simulink model "skipper_lqr"  (R2024b)
settings: Solver=FixedStepAuto  StartTime=0.0  StopTime=20  RelTol=1e-3
libraries: matrix_library x2, aerolibanimutils x1, dspinverses x1
settings Model: Creator=nehir  LastModifiedBy=nehir
settings OptimizationCC: OptimizeBlockIOStorage=off  OptimizeDataStoreBuffers=off  BusAssignmentInplaceUpdate=off
settings DebuggingCC: SFUnexpectedBacktrackingDiag=warning  SFNoUnconditionalDefaultTransitionDiag=warning
settings RTWCC: GenerateReport=on  BuildConfiguration=Debug  LaunchReport=on
settings CodeAppCC: ForceParamTrailComments=on  MATLABSourceComments=on  EnableCustomComments=on
settings GRTTargetCC: CombineSignalStateStructs=on  SupportVariableSizeSignals=on  MultiInstanceErrorCode=Warning

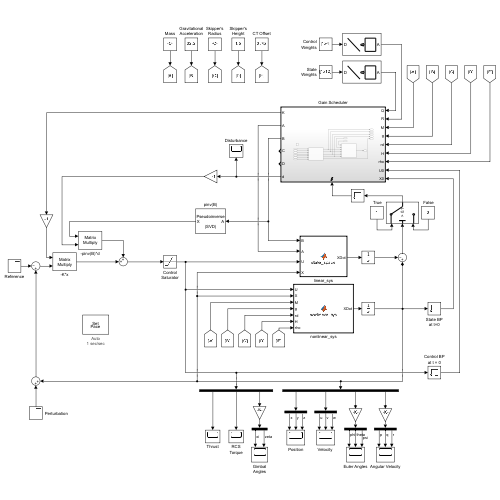
[thumbnail: Simulink's stored preview of the top-level diagram]
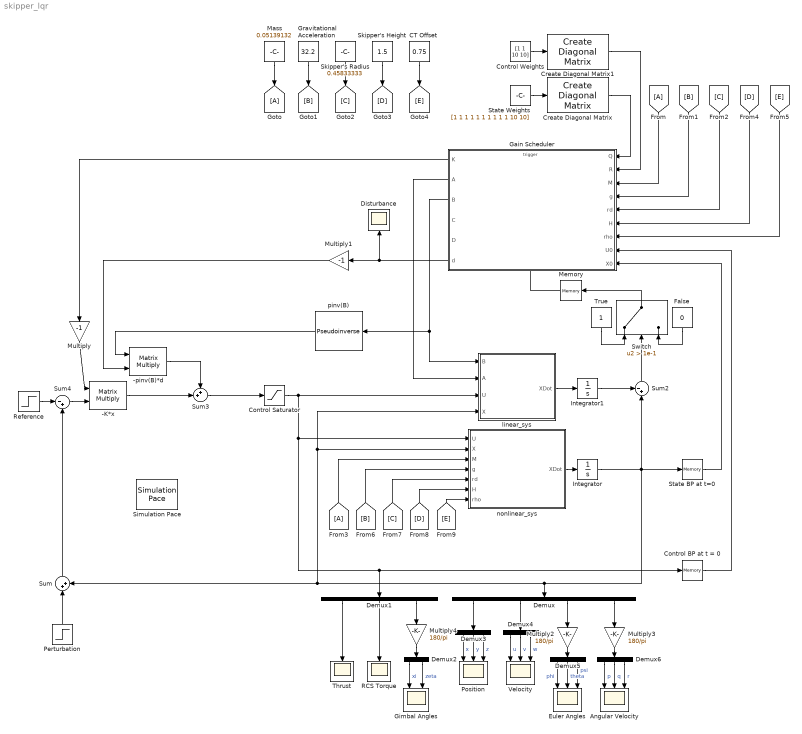
== system skipper_lqr ==
  " False" : Constant  Value=0
  " True" : Constant
  -K*x : Product  Multiplication=Matrix(*)
  -pinv(B)*d : Product  Multiplication=Matrix(*)
  Angular Velocity : Scope  NumInputPorts=3
  CT Offset : Constant  Value=0.75
  Control Saturator : Saturate  UpperLimit=[2.2 pi/2 pi/18 pi/18]'  LowerLimit=[0 -pi/2 -pi/18 -pi/18]'
  Control Weights : Constant  Value=[1 1 10 10]
  Control BP at t = 0 : Memory  InitialCondition=[10 1 0 0]'
  Create Diagonal Matrix : matrix_library/Create Diagonal Matrix
      settings: LibrarySourceBlock=|
      | simulink/Matrix
      | Operations/Create Diagonal
      | Matrix
  Create Diagonal Matrix1 : matrix_library/Create Diagonal Matrix
      settings: LibrarySourceBlock=|
      | simulink/Matrix
      | Operations/Create Diagonal
      | Matrix
  Demux : Demux  Outputs=[3 3 3 3]
  Demux1 : Demux  Outputs=[1 1 2]
  Demux2 : Demux  Outputs=[1 1]
  Demux{3..6} (4 alike) : Demux  Outputs=[1 1 1]
  Disturbance : Scope
  Euler Angles : Scope  NumInputPorts=3
  From : From
  From3 : From
  Gain Scheduler : Subsystem  TreatAsAtomicUnit=on
  Gimbal Angles : Scope  NumInputPorts=2
  Goto : Goto
  Gravitational Acceleration : Constant  Value=32.2
  Integrator : Integrator  InitialCondition=[0 0 0 0 0 0 0 0 0 0 0 0]'
  Integrator1 : Integrator  InitialCondition=[0 0 0 0 0 0 0 0 0 0 0 0]'
  Mass : Constant  Value=0.05139132
  Memory : Memory  InitialCondition=1
  Multiply : Gain  Gain=-1
  Multiply1 : Gain  Gain=-1
  Multiply2 : Gain  Gain=180/pi
  Multiply3 : Gain  Gain=180/pi
  Multiply4 : Gain  Gain=180/pi
  Perturbation : Step  Time=0.1  Before=[0 0 0 0 0 0 0 0 0 0 0 0]'  After=[0 0 0 0 0 0 0 0 0 0 0 0]'  SampleTime=0
  Position : Scope  NumInputPorts=3
  RCS Torque : Scope
  Reference : Step  Before=[0 0 0 0 0 0 0 0 0 0 0 0]'  After=[5 5 5 0 0 0 0 0 0 0 0 0]'  SampleTime=0
  Simulation Pace : aerolibanimutils/Simulation Pace  SimulationPace=1  SleepMode=Auto  OutputPaceError=off  SampleTime=1/30
  Skipper's Height : Constant  Value=1.5
  Skipper's Radius : Constant  Value=0.45833333
  State Weights : Constant  Value=[1 1 1 1 1 1 1 1 1 1 10 10]
  State BP at t=0 : Memory  InitialCondition=[0 0 0 0 0 0 0 0 0 0 0 0]'
  Sum : Sum  Inputs=|++
  Sum2 : Sum  Inputs=-+|
  Sum3 : Sum  Inputs=++|
  Sum4 : Sum  Inputs=|-+
  Switch : Switch  Criteria=u2 > Threshold  Threshold=1e-1  ZeroCross=off  SaturateOnIntegerOverflow=off  InputSameDT=off
  Thrust : Scope
  "Velocity " : Scope  NumInputPorts=3
  linear_sys : MATLAB Function  TreatAsAtomicUnit=on
  nonlinear_sys : MATLAB Function  TreatAsAtomicUnit=on
  pinv(B) : dspinverses/Pseudoinverse  wanterr=off  SimulateUsing=Interpreted execution
  wires:
  Demux1/2 -> RCS Torque/1
  Demux1/1 -> Thrust/1
  Demux/1 -> Demux3/1
  Demux/2 -> Demux4/1
  Demux/3 -> Multiply2/1
  Demux/4 -> Multiply3/1
  Demux1/3 -> Multiply4/1
  Demux2/1 -> Gimbal Angles/1  "xi"
  Demux2/2 -> Gimbal Angles/2  "zeta"
  Demux3/1 -> Position/1  "x"
  Demux3/3 -> Position/3  "z"
  Demux4/1 -> "Velocity "/1  "u"
  Demux4/2 -> "Velocity "/2  "v"
  Demux4/3 -> "Velocity "/3  "w"
  Demux5/1 -> Euler Angles/1  "phi"
  Demux5/2 -> Euler Angles/2  "theta"
  Demux5/3 -> Euler Angles/3  "psi"
  Demux3/2 -> Position/2  "y"
  Demux6/1 -> Angular Velocity/1  "p"
  Demux6/2 -> Angular Velocity/2  "q"
  Demux6/3 -> Angular Velocity/3  "r"
  nonlinear_sys/1(XDot) -> Integrator/1
  Sum4/1 -> -K*x/2
  Sum2/1 -> Switch/2
  linear_sys/1(XDot) -> Integrator1/1
  Integrator1/1 -> Sum2/1
  State Weights/1 -> Create Diagonal Matrix/1
  Control Weights/1 -> Create Diagonal Matrix1/1
  Multiply/1 -> -K*x/1
  pinv(B)/1 -> -pinv(B)*d/1
  Multiply1/1 -> -pinv(B)*d/2
  Gain Scheduler/6(d) -> Disturbance/1, Multiply1/1
  Gain Scheduler/3(B) -> pinv(B)/1, linear_sys/1(B)
  Gain Scheduler/1(K) -> Multiply/1
  Switch/1 -> Memory/1
  " True"/1 -> Switch/1
  " False"/1 -> Switch/3
  Create Diagonal Matrix/1 -> Gain Scheduler/1(Q)
  Create Diagonal Matrix1/1 -> Gain Scheduler/2(R)
  Gain Scheduler/2(A) -> linear_sys/2(A)
  Integrator/1 -> Demux/1, nonlinear_sys/2(X), linear_sys/4(X), Sum/2, State BP at t=0/1, Sum2/2
  Control BP at t = 0/1 -> Gain Scheduler/8(U0)
  State BP at t=0/1 -> Gain Scheduler/9(X0)
  Memory/1 -> Gain Scheduler/Trigger
  -K*x/1 -> Sum3/2
  Control Saturator/1 -> linear_sys/3(U), nonlinear_sys/1(U), Demux1/1, Control BP at t = 0/1
  Multiply2/1 -> Demux5/1
  Multiply3/1 -> Demux6/1
  Multiply4/1 -> Demux2/1
  [E] -> nonlinear_sys/7(rho)
  [B] -> nonlinear_sys/4(g)
  [D] -> nonlinear_sys/6(H)
  [C] -> nonlinear_sys/5(rd)
  From3/1 -> nonlinear_sys/3(M)
  CT Offset/1 -> [E]
  Gravitational Acceleration/1 -> [B]
  Mass/1 -> Goto/1
  Skipper's Height/1 -> [D]
  Skipper's Radius/1 -> [C]
  [D] -> Gain Scheduler/6(H)
  [B] -> Gain Scheduler/4(g)
  [C] -> Gain Scheduler/5(rd)
  From/1 -> Gain Scheduler/3(M)
  [E] -> Gain Scheduler/7(rho)
  Reference/1 -> Sum4/1
  Sum/1 -> Sum4/2
  Perturbation/1 -> Sum/1
  Sum3/1 -> Control Saturator/1
  -pinv(B)*d/1 -> Sum3/1

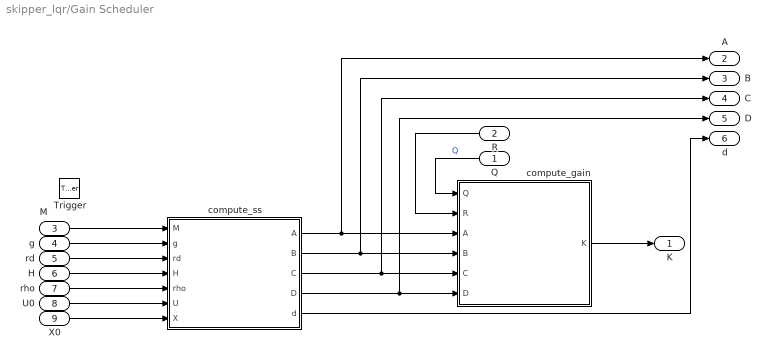
== system skipper_lqr/Gain Scheduler ==
  Q : Inport
  R : Inport  Port=2
  M : Inport  Port=3
  g : Inport  Port=4
  rd : Inport  Port=5
  H : Inport  Port=6
  rho : Inport  Port=7
  U0 : Inport  Port=8
  X0 : Inport  Port=9
  Trigger : TriggerPort  VariantControl=(inherit)  ZeroCross=off  InitialTriggerSignalState=negative
  compute_gain : MATLAB Function  TreatAsAtomicUnit=on
  compute_ss : MATLAB Function  TreatAsAtomicUnit=on
  K : Outport
  A : Outport  Port=2
  B : Outport  Port=3
  C : Outport  Port=4
  D : Outport  Port=5
  d : Outport  Port=6
  wires:
  M/1 -> compute_ss/1(M)
  R/1 -> compute_gain/2(R)
  Q/1 -> compute_gain/1(Q)  "Q"
  U0/1 -> compute_ss/6(U)
  rho/1 -> compute_ss/5(rho)
  H/1 -> compute_ss/4(H)
  rd/1 -> compute_ss/3(rd)
  g/1 -> compute_ss/2(g)
  X0/1 -> compute_ss/7(X)
  compute_ss/1(A) -> A/1, compute_gain/3(A)
  compute_ss/2(B) -> B/1, compute_gain/4(B)
  compute_ss/3(C) -> compute_gain/5(C), C/1
  compute_ss/4(D) -> compute_gain/6(D), D/1
  compute_ss/5(d) -> d/1
  compute_gain/1(K) -> K/1

== matlab function skipper_lqr/Gain Scheduler/compute_ss ==
  data: M input; g input; rd input; H input; rho input; U input; X input; A output; B output; C output; D output; d output
function [A, B, C, D, d] = compute_ss(M, g, rd, H, rho, U, X)
% ________________________________________________________________________
%
%                           STATE SPACE MATRICES
% ________________________________________________________________________
% 
% BY:       FLORIDA ROCKET LAB - GNC SUBTEAM
% EDITORS:  N. HIRSCH, L. DAPP
% DATE:     1/20/25
%
% OVERVIEW: Calculates A, B, C, D, matices for use in a state
% space Simulink model and LQR controller as well as the disturbance, d.

    %save('basepoints.mat', 'U', 'X')
    
    % Calculate rotational inertias in body frame.
    Ixx = M*rd^2/2;
    Iyy = M*(3*rd^2+H^2)/12;
    Izz = Iyy;
    
    % Initialize state space matricies. Since they are sparse simply use zeros
    % and then input non-zero terms individually.
    % x = [x y z u v w phi theta psi p q r]
    % u = [T tauR xi zeta]
    x0 = X(1);
    y0 = X(2);
    z0 = X(3);
    u0 = X(4);
    v0 = X(5);
    w0 = X(6);
    phi0 = X(7);
    theta0 = X(8);
    psi0 = X(9);
    p0 = X(10);
    q0 = X(11);
    r0 = X(12);

    T0 = U(1);
    tauR0 = U(2);
    xi0 = U(3);
    zeta0 = U(4);

    % BEGIN "A"; Do not modify this. The python script looks for this line.
    A = [
        0 0 0 cos(psi0)*cos(theta0) sin(phi0)*sin(theta0)*cos(psi0)-sin(psi0)*cos(phi0) sin(phi0)*sin(psi0)+sin(theta0)*cos(phi0)*cos(psi0) v0*sin(phi0)*sin(psi0)+v0*sin(theta0)*cos(phi0)*cos(psi0)-w0*sin(phi0)*sin(theta0)*cos(psi0)+w0*sin(psi0)*cos(phi0) -u0*sin(theta0)*cos(psi0)+v0*sin(phi0)*cos(psi0)*cos(theta0)+w0*cos(phi0)*cos(psi0)*cos(theta0) -u0*sin(psi0)*cos(theta0)-v0*sin(phi0)*sin(psi0)*sin(theta0)-v0*cos(phi0)*cos(psi0)+w0*sin(phi0)*cos(psi0)-w0*sin(psi0)*sin(theta0)*cos(phi0) 0 0 0;
        0 0 0 sin(psi0)*cos(theta0) sin(phi0)*sin(psi0)*sin(theta0)+cos(phi0)*cos(psi0) -sin(phi0)*cos(psi0)+sin(psi0)*sin(theta0)*cos(phi0) -v0*sin(phi0)*cos(psi0)+v0*sin(psi0)*sin(theta0)*cos(phi0)-w0*sin(phi0)*sin(psi0)*sin(theta0)-w0*cos(phi0)*cos(psi0) -u0*sin(psi0)*sin(theta0)+v0*sin(phi0)*sin(psi0)*cos(theta0)+w0*sin(psi0)*cos(phi0)*cos(theta0) u0*cos(psi0)*cos(theta0)+v0*sin(phi0)*sin(theta0)*cos(psi0)-v0*sin(psi0)*cos(phi0)+w0*sin(phi0)*sin(psi0)+w0*sin(theta0)*cos(phi0)*cos(psi0) 0 0 0;
        0 0 0 -sin(theta0) sin(phi0)*cos(theta0) cos(phi0)*cos(theta0) v0*cos(phi0)*cos(theta0)-w0*sin(phi0)*cos(theta0) -u0*cos(theta0)-v0*sin(phi0)*sin(theta0)-w0*sin(theta0)*cos(phi0) 0 0 0 0;
        0 0 0 0 r0 -q0 0 g*sin(theta0)*cos(psi0) g*sin(psi0)*cos(theta0) 0 -w0 v0;
        0 0 0 -r0 0 p0 -g*sin(phi0)*sin(psi0)-g*sin(theta0)*cos(phi0)*cos(psi0) -g*sin(phi0)*cos(psi0)*cos(theta0) g*sin(phi0)*sin(psi0)*sin(theta0)+g*cos(phi0)*cos(psi0) w0 0 -u0;
        0 0 0 q0 -p0 0 g*sin(phi0)*sin(theta0)*cos(psi0)-g*sin(psi0)*cos(phi0) -g*cos(phi0)*cos(psi0)*cos(theta0) -g*sin(phi0)*cos(psi0)+g*sin(psi0)*sin(theta0)*cos(phi0) -v0 u0 0;
        0 0 0 0 0 0 q0*cos(phi0)*tan(theta0)-r0*sin(phi0)*tan(theta0) q0*sin(phi0)*tan(theta0)^2+q0*sin(phi0)+r0*cos(phi0)*tan(theta0)^2+r0*cos(phi0) 0 1 sin(phi0)*tan(theta0) cos(phi0)*tan(theta0);
        0 0 0 0 0 0 -q0*sin(phi0)-r0*cos(phi0) 0 0 0 cos(phi0) -sin(phi0);
        0 0 0 0 0 0 q0*cos(phi0)/cos(theta0)-r0*sin(phi0)/cos(theta0) q0*sin(phi0)*sin(theta0)/cos(theta0)^2+r0*sin(theta0)*cos(phi0)/cos(theta0)^2 0 0 sin(phi0)/cos(theta0) cos(phi0)/cos(theta0);
        0 0 0 0 0 0 0 0 0 0 Iyy*r0/Ixx-Izz*r0/Ixx Iyy*q0/Ixx-Izz*q0/Ixx;
        0 0 0 0 0 0 0 0 0 -Ixx*r0/Iyy+Izz*r0/Iyy 0 -Ixx*p0/Iyy+Izz*p0/Iyy;
        0 0 0 0 0 0 0 0 0 Ixx*q0/Izz-Iyy*q0/Izz Ixx*p0/Izz-Iyy*p0/Izz 0;
    ];
    % END "A"; Do not modify this. The python script looks for this line.

    % u = [T tauR xi zeta]

    % BEGIN "B"; Do not modify this. The python script looks for this line.
    B = [
        0 0 0 0;
        0 0 0 0;
        0 0 0 0;
        cos(xi0)*cos(zeta0)/M 0 -T0*sin(xi0)*cos(zeta0)/M -T0*sin(zeta0)*cos(xi0)/M;
        sin(zeta0)/M 0 0 T0*cos(zeta0)/M;
        -sin(xi0)*cos(zeta0)/M 0 -T0*cos(xi0)*cos(zeta0)/M T0*sin(xi0)*sin(zeta0)/M;
        0 0 0 0;
        0 0 0 0;
        0 0 0 0;
        0 1/Ixx 0 0;
        -rho*sin(xi0)*cos(zeta0)/Iyy 0 -T0*rho*cos(xi0)*cos(zeta0)/Iyy T0*rho*sin(xi0)*sin(zeta0)/Iyy;
        -rho*sin(zeta0)/Izz 0 0 -T0*rho*cos(zeta0)/Izz;
    ];
    % END "B"; Do not modify this. The python script looks for this line.

   % BEGIN "d"; Do not modify this. The python script looks for this line.
    d = [
        -phi0*v0*sin(phi0)*sin(psi0) - phi0*v0*sin(theta0)*cos(phi0)*cos(psi0) + phi0*w0*sin(phi0)*sin(theta0)*cos(psi0) - phi0*w0*sin(psi0)*cos(phi0) + psi0*u0*sin(psi0)*cos(theta0) + psi0*v0*sin(phi0)*sin(psi0)*sin(theta0) + psi0*v0*cos(phi0)*cos(psi0) - psi0*w0*sin(phi0)*cos(psi0) + psi0*w0*sin(psi0)*sin(theta0)*cos(phi0) + theta0*u0*sin(theta0)*cos(psi0) - theta0*v0*sin(phi0)*cos(psi0)*cos(theta0) - theta0*w0*cos(phi0)*cos(psi0)*cos(theta0);
        phi0*v0*sin(phi0)*cos(psi0) - phi0*v0*sin(psi0)*sin(theta0)*cos(phi0) + phi0*w0*sin(phi0)*sin(psi0)*sin(theta0) + phi0*w0*cos(phi0)*cos(psi0) - psi0*u0*cos(psi0)*cos(theta0) - psi0*v0*sin(phi0)*sin(theta0)*cos(psi0) + psi0*v0*sin(psi0)*cos(phi0) - psi0*w0*sin(phi0)*sin(psi0) - psi0*w0*sin(theta0)*cos(phi0)*cos(psi0) + theta0*u0*sin(psi0)*sin(theta0) - theta0*v0*sin(phi0)*sin(psi0)*cos(theta0) - theta0*w0*sin(psi0)*cos(phi0)*cos(theta0);
        -phi0*v0*cos(phi0)*cos(theta0) + phi0*w0*sin(phi0)*cos(theta0) + theta0*u0*cos(theta0) + theta0*v0*sin(phi0)*sin(theta0) + theta0*w0*sin(theta0)*cos(phi0);
        -g*psi0*sin(psi0)*cos(theta0) - g*theta0*sin(theta0)*cos(psi0) - g*cos(psi0)*cos(theta0) + q0*w0 - r0*v0 + T0*xi0*sin(xi0)*cos(zeta0)/M + T0*zeta0*sin(zeta0)*cos(xi0)/M;
        g*phi0*sin(phi0)*sin(psi0) + g*phi0*sin(theta0)*cos(phi0)*cos(psi0) - g*psi0*sin(phi0)*sin(psi0)*sin(theta0) - g*psi0*cos(phi0)*cos(psi0) + g*theta0*sin(phi0)*cos(psi0)*cos(theta0) - g*sin(phi0)*sin(theta0)*cos(psi0) + g*sin(psi0)*cos(phi0) - p0*w0 + r0*u0 - T0*zeta0*cos(zeta0)/M;
        -g*phi0*sin(phi0)*sin(theta0)*cos(psi0) + g*phi0*sin(psi0)*cos(phi0) + g*psi0*sin(phi0)*cos(psi0) - g*psi0*sin(psi0)*sin(theta0)*cos(phi0) + g*theta0*cos(phi0)*cos(psi0)*cos(theta0) - g*sin(phi0)*sin(psi0) - g*sin(theta0)*cos(phi0)*cos(psi0) + p0*v0 - q0*u0 + T0*xi0*cos(xi0)*cos(zeta0)/M - T0*zeta0*sin(xi0)*sin(zeta0)/M;
        -phi0*q0*cos(phi0)*tan(theta0) + phi0*r0*sin(phi0)*tan(theta0) - q0*theta0*sin(phi0)*tan(theta0)^2 - q0*theta0*sin(phi0) - r0*theta0*cos(phi0)*tan(theta0)^2 - r0*theta0*cos(phi0);
        phi0*q0*sin(phi0) + phi0*r0*cos(phi0);
        -phi0*q0*cos(phi0)/cos(theta0) + phi0*r0*sin(phi0)/cos(theta0) - q0*theta0*sin(phi0)*sin(theta0)/cos(theta0)^2 - r0*theta0*sin(theta0)*cos(phi0)/cos(theta0)^2;
        -Iyy*q0*r0/Ixx + Izz*q0*r0/Ixx;
        Ixx*p0*r0/Iyy - Izz*p0*r0/Iyy + T0*rho*xi0*cos(xi0)*cos(zeta0)/Iyy - T0*rho*zeta0*sin(xi0)*sin(zeta0)/Iyy;
        -Ixx*p0*q0/Izz + Iyy*p0*q0/Izz + T0*rho*zeta0*cos(zeta0)/Izz;
    ];
    % END "d"; Do not modify this. The python script looks for this line.
   
    C = diag(ones(1, 12));
    
    D = zeros(size(B));
end

== matlab function skipper_lqr/linear_sys ==
  data: B input; A input; U input; XDot output; X input
function XDot = state_space(B, A, U, X)
    XDot = A*X + B*U;
end

== matlab function skipper_lqr/Gain Scheduler/compute_gain ==
  data: Q input; R input; A input; K output; B input; C input; D input
function K = compute_gain(Q, R, A, B, C, D)
    
    %care = @(S) A'*S + S*A - S*B*inv(R)*B'*S + Q;
    %S0 = zeros(size(A, 1), size(A, 2));
    %options = optimoptions('lsqnonlin', 'Algorithm', 'levenberg-marquardt');
    %S = lsqnonlin(care, S0, [], [], options);
    %K = inv(R)*B'*S;

    %coder.extrinsic('icare')
    K = zeros(4, 12);
    %[~, K] = icare(A, B, Q, R);

end

== matlab function skipper_lqr/nonlinear_sys ==
  data: U input; XDot output; X input; M input; g input; rd input; H input; rho input
function XDot = nonlinear_sys(U, X, M, g, rd, H, rho)
    
    Ixx = M*rd^2/2;
    Iyy = M*(3*rd^2+H^2)/12;
    Izz = Iyy;

    x = X(1);
    y = X(2);
    z = X(3);
    u = X(4);
    v = X(5);
    w = X(6);
    phi = X(7);
    theta = X(8);
    psi = X(9);
    p = X(10);
    q = X(11);
    r = X(12);

    T = U(1);
    tauR = U(2);
    xi = U(3);
    zeta = U(4);

    xDot = w*(sin(phi)*sin(psi) + cos(phi)*cos(psi)*sin(theta)) - v*(cos(phi)*sin(psi) - cos(psi)*sin(phi)*sin(theta)) + u*cos(psi)*cos(theta);
    yDot = v*(cos(phi)*cos(psi) + sin(phi)*sin(psi)*sin(theta)) - w*(cos(psi)*sin(phi) - cos(phi)*sin(psi)*sin(theta)) + u*cos(theta)*sin(psi);
    zDot = w*cos(phi)*cos(theta) - u*sin(theta) + v*cos(theta)*sin(phi);
    uDot = (T*cos(xi)*cos(zeta) - M*q*w + M*r*v - M*g*cos(psi)*cos(theta))/M;
    vDot = (T*sin(zeta) + M*p*w - M*r*u + M*g*cos(phi)*sin(psi) - M*g*cos(psi)*sin(phi)*sin(theta))/M;
    wDot = -(T*cos(zeta)*sin(xi) + M*p*v - M*q*u + M*g*sin(phi)*sin(psi) + M*g*cos(phi)*cos(psi)*sin(theta))/M;
    phiDot = p + r*cos(phi)*tan(theta) + q*sin(phi)*tan(theta);
    thetaDot = q*cos(phi) - r*sin(phi);
    psiDot = (r*cos(phi))/cos(theta) + (q*sin(phi))/cos(theta);
    pDot = (tauR + Iyy*q*r - Izz*q*r)/Ixx;
    qDot = -(Ixx*p*r - Izz*p*r + T*rho*cos(zeta)*sin(xi))/Iyy;
    rDot = -(T*rho*sin(zeta) - Ixx*p*q + Iyy*p*q)/Izz;

    XDot = [xDot yDot zDot uDot vDot wDot phiDot thetaDot psiDot pDot qDot rDot]';
end
